simulink model "adarbha_hw6_sim"  (Simulink 7.7)
settings: Solver=ode1  StartTime=0.0  StopTime=max(Time)  FixedStep=0.5  RelTol=1e-5
InitFcn:
  | adarbha_hw6
values from neighbouring files (symbols this model uses):
  Area = 2.7    [adarbha_hw6.m]    (also in hw6.m; hw6_code.m)
  Cd = 0.44    [adarbha_hw6.m]    (also in hw6.m; hw6_code.m)
  density = 1.224    [adarbha_hw6.m]    (also in hw6.m; hw6_code.m)
  Q = 20    [adarbha_hw6.m]    (also in hw6_code.m)
  R_batt = 0.1    [adarbha_hw6.m]    (also in hw6_code.m)
  radius_wheel_m = 0.41    [adarbha_hw6.m]    (also in hw6.m; hw6_code.m)
  rpm = 1:5000    [adarbha_hw6.m]    (also in hw6.m; hw6_code.m)
  Time = xlsread('Malibu_20100929_highway_Baseline','A:A')    [adarbha_hw6.m]    (also in hw6.m; hw6_code.m)
  time_s = time_scale*100    [adarbha_hw6.m]    (also in hw6.m; hw6_code.m)
  V_o = 300    [adarbha_hw6.m]    (also in hw6_code.m)
  vel_m_s = M_number*3    [adarbha_hw6.m]    (also in hw6.m; hw6_code.m)
  Velocity_kph = xlsread('Malibu_20100929_highway_Baseline','B:B')    [adarbha_hw6.m]    (also in hw6.m; hw6_code.m)
  weight_N = 16000    [adarbha_hw6.m]    (also in hw6.m; hw6_code.m)
undefined symbols (not defined in the file or in its folder): torque
libraries: simulink x3
settings Model: Creator=Arjun  LastModifiedBy=Arjun
settings DataIOCC: SignalLogging=off
settings DebuggingCC: AlgebraicLoopMsg=none

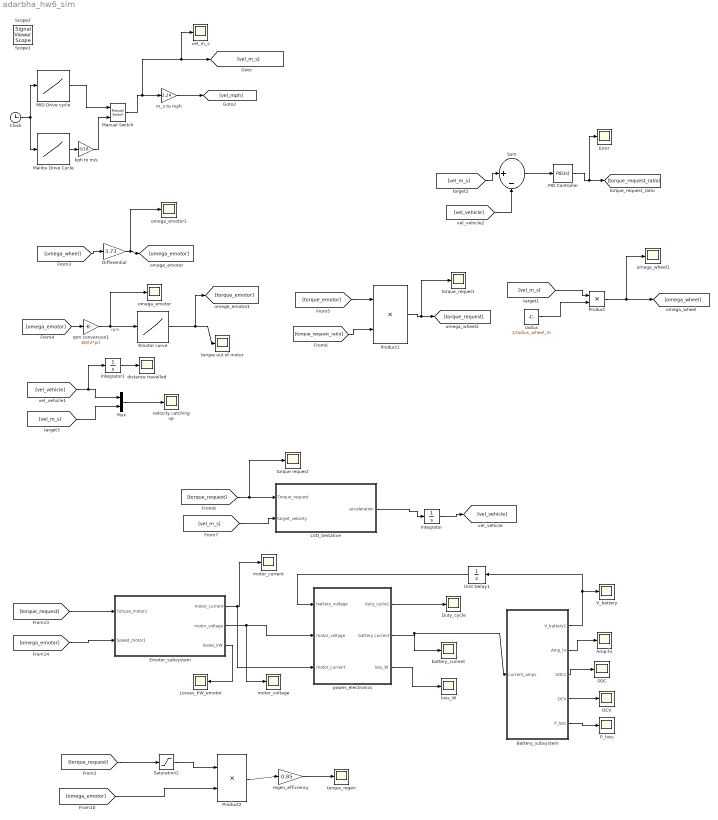
== system adarbha_hw6_sim ==
  note: rpm
  Amp-hr : Scope
      settings: SaveName=ScopeData23
  Battery_subsystem : Subsystem
  Clock : Clock
      settings: Decimation=10
  Differential : Gain  Gain=3.73
  Duty_cycle : Scope
      settings: SaveName=ScopeData22
  Emotor curve : Lookup_n-D  NumberOfTableDimensions=1  BreakpointsForDimension1=rpm  Table=torque  RndMeth=Simplest  InputSameDT=on
  Emotor_subsystem : Subsystem
  Error : Scope
      settings: SaveName=ScopeData17
  Integrator : Integrator
  Integrator1 : Integrator
  LVD_tentative : Subsystem
  Losses_kW_emotor : Scope
      settings: SaveName=ScopeData19
  MID Drive cycle : Lookup_n-D  NumberOfTableDimensions=1  BreakpointsForDimension1=time_s  Table=vel_m_s  RndMeth=Simplest  InputSameDT=on
  Malibu Drive Cycle : Lookup_n-D  NumberOfTableDimensions=1  BreakpointsForDimension1=Time  Table=Velocity_kph  RndMeth=Simplest  InputSameDT=on
  Manual Switch : simulink/Signal Routing/Manual Switch  SystemSampleTime=-1  sw=0  action=0  varsize=off
  Mux : Mux  Inputs=2
  OCV : Scope
      settings: SaveName=ScopeData31
  PID Controller : simulink/Continuous/PID Controller  SystemSampleTime=-1  Controller=PID  TimeDomain=Continuous-time  SampleTime=1  IntegratorMethod=Forward Euler  FilterMethod=Forward Euler  Form=Parallel  P=1  I=1  D=0  N=100  InitialConditionSource=internal  InitialConditionForIntegrator=0  InitialConditionForFilter=0  ExternalReset=none  LimitOutput=off  UpperSaturationLimit=inf  LowerSaturationLimit=-inf  LinearizeAsGain=off  AntiWindupMode=none  Kb=1  TrackingMode=off  Kt=1  PParamMin=[]  PParamMax=[]  IParamMin=[]  IParamMax=[]  DParamMin=[]  DParamMax=[]  NParamMin=[]  NParamMax=[]  KbParamMin=[]  KbParamMax=[]  KtParamMin=[]  KtParamMax=[]  POutMin=[]  POutMax=[]  IOutMin=[]  IOutMax=[]  DOutMin=[]  DOutMax=[]  NOutMin=[]  NOutMax=[]  KbOutMin=[]  KbOutMax=[]  KtOutMin=[]  KtOutMax=[]  IntegratorOutMin=[]  IntegratorOutMax=[]  FilterOutMin=[]  FilterOutMax=[]  SumOutMin=[]  SumOutMax=[]  SumI1OutMin=[]  SumI1OutMax=[]  SumI2OutMin=[]  SumI2OutMax=[]  SumI3OutMin=[]  SumI3OutMax=[]  SumDOutMin=[]  SumDOutMax=[]  SaturationOutMin=[]  SaturationOutMax=[]  IntegratorContinuousStateAttributes=''  IntegratorStateMustResolveToSignalObject=off  IntegratorRTWStateStorageClass=Auto  FilterContinuousStateAttributes=''  FilterStateMustResolveToSignalObject=off  FilterRTWStateStorageClass=Auto
  P_loss : Scope
      settings: SaveName=ScopeData33
  Product : Product  RndMeth=Zero
  Product1 : Product  RndMeth=Zero
  Product2 : Product  RndMeth=Zero
  SOC : Scope
      settings: SaveName=ScopeData28
  Saturation2 : Saturate  UpperLimit=0  LowerLimit=-Inf
  Sum : Sum  Inputs=|+-
  Unit Delay1 : UnitDelay  SampleTime=-1
  V_battery : Scope
      settings: TimeRange=500  YMin=-50  YMax=300  SaveName=ScopeData29
  battery_current : Scope
      settings: SaveName=ScopeData24
  distance travelled : Scope
      settings: SaveName=ScopeData25
  kph to m/s : Gain  Gain=5/18
  loss_W : Scope
      settings: SaveName=ScopeData20
  m_s to mph : Gain  Gain=2.24
  motor_current : Scope
      settings: SaveName=ScopeData11
  motor_voltage : Scope
      settings: SaveName=ScopeData26
  omega_emotor : Scope
      settings: SaveName=ScopeData7
  omega_emotor1 : Scope
      settings: SaveName=ScopeData32
  omega_wheel1 : Scope
      settings: SaveName=ScopeData4
  power_electronics : Subsystem
  radius : Constant  Value=1/radius_wheel_m
  regen_efficiency : Gain  Gain=0.85
  rpm conversion1 : Gain  Gain=60/(2*pi)
  torque out of motor : Scope
      settings: SaveName=ScopeData8
  torque request : Scope
      settings: SaveName=ScopeData12
  torque_regen : Scope
      settings: SaveName=ScopeData16
  torque_request : Scope
      settings: SaveName=ScopeData6
  vel_m_s : Scope
      settings: SaveName=ScopeData21
  velocity catching up : Scope
      settings: TimeRange=765.8724058416602  YMin=-1e+049  YMax=9.000000000000001e+049  SaveName=ScopeData18
  Scope1 : SignalViewerScope  IOType=viewer  NumInputPorts=5  RefreshTime=0.035000
  Scope2 : SignalViewerScope  IOType=viewer  RefreshTime=0.035000
  wires:
  m_s to mph/1 -> [vel_mph]
  Clock/1 -> MID Drive cycle/1, Malibu Drive Cycle/1
  [vel_m_s] -> Product/1
  Product/1 -> [omega_wheel], omega_wheel1/1
  radius/1 -> Product/2
  [torque_emotor] -> Product1/1
  [torque_request_ratio] -> Product1/2
  Product1/1 -> [torque_request], torque_request/1
  [omega_wheel] -> Differential/1
  Differential/1 -> [omega_emotor], omega_emotor1/1
  [omega_emotor] -> rpm conversion1/1
  Emotor curve/1 -> torque out of motor/1, [torque_emotor]
  [vel_m_s] -> LVD_tentative/2(target_velocity)
  [torque_request] -> LVD_tentative/1(Torque_request), torque request/1
  Integrator/1 -> [vel_vehicle]
  LVD_tentative/1(acceleration) -> Integrator/1
  [vel_m_s] -> Sum/1
  [vel_vehicle] -> Sum/2
  [vel_m_s] -> Mux/2
  [vel_vehicle] -> Mux/1, Integrator1/1
  Mux/1 -> velocity catching up/1
  MID Drive cycle/1 -> Manual Switch/1
  Manual Switch/1 -> m_s to mph/1, [vel_m_s], vel_m_s/1
  Malibu Drive Cycle/1 -> kph to m/s/1
  kph to m/s/1 -> Manual Switch/2
  Integrator1/1 -> distance travelled/1
  power_electronics/2(battery current) -> battery_current/1, Battery_subsystem/1(current_amps)
  Battery_subsystem/1(V_battery1) -> V_battery/1, Unit Delay1/1
  Battery_subsystem/3(SOC1) -> SOC/1
  [torque_request] -> Saturation2/1
  Saturation2/1 -> Product2/1
  [omega_emotor] -> Product2/2
  Product2/1 -> regen_efficiency/1
  regen_efficiency/1 -> torque_regen/1
  power_electronics/3(loss_W) -> loss_W/1
  power_electronics/1(duty_cycle1) -> Duty_cycle/1
  Battery_subsystem/2(Amp_hr) -> Amp-hr/1
  Battery_subsystem/4(OCV) -> OCV/1
  Battery_subsystem/5(P_loss) -> P_loss/1
  rpm conversion1/1 -> Emotor curve/1, omega_emotor/1
  Unit Delay1/1 -> power_electronics/1(battery_voltage)
  Emotor_subsystem/3(losses_kW) -> Losses_kW_emotor/1
  Emotor_subsystem/2(motor_voltage) -> power_electronics/2(motor_voltage), motor_voltage/1
  Emotor_subsystem/1(motor_current) -> motor_current/1, power_electronics/3(motor_current)
  [torque_request] -> Emotor_subsystem/1(Torque_motor1)
  [omega_emotor] -> Emotor_subsystem/2(Speed_motor1)
  Sum/1 -> PID Controller/1
  PID Controller/1 -> [torque_request_ratio], Error/1

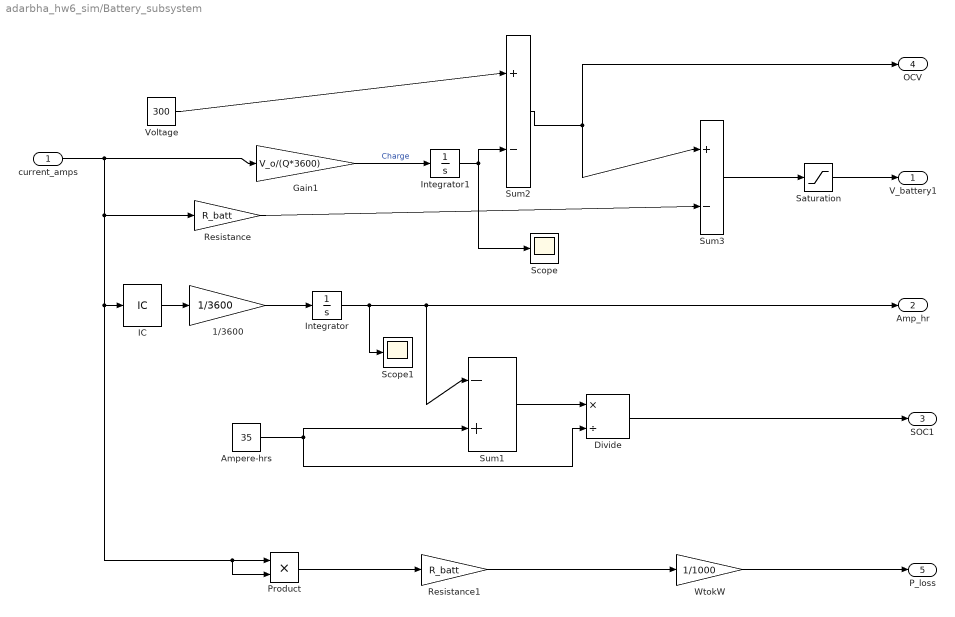
== system adarbha_hw6_sim/Battery_subsystem ==
  current_amps : Inport
  1/3600 : Gain  Gain=1/3600
  Ampere-hrs : Constant  Value=35
  Divide : Product  Inputs=*/
  Gain1 : Gain  Gain=V_o/(Q*3600)
  IC : InitialCondition  Value=0.1
  Integrator : Integrator  InitialCondition=0.1  LimitOutput=on  UpperSaturationLimit=20  LowerSaturationLimit=0
  Integrator1 : Integrator  LimitOutput=on  UpperSaturationLimit=300  LowerSaturationLimit=0
  Product : Product  RndMeth=Zero
  Resistance : Gain  Gain=R_batt
  Resistance1 : Gain  Gain=R_batt
  Saturation : Saturate  UpperLimit=300  LowerLimit=1  ZeroCross=off
  Scope : Scope
  Scope1 : Scope
      settings: SaveName=ScopeData3
  Sum1 : Sum  Inputs=|-+
  Sum2 : Sum  Inputs=|+-
  Sum3 : Sum  Inputs=|+-
  Voltage : Constant  Value=300
  WtokW : Gain  Gain=1/1000
  V_battery1 : Outport
  Amp_hr : Outport  Port=2
  SOC1 : Outport  Port=3
  OCV : Outport  Port=4
  P_loss : Outport  Port=5
  wires:
  Gain1/1 -> Integrator1/1  "Charge"
  Integrator1/1 -> Sum2/2, Scope/1
  Resistance/1 -> Sum3/2
  Ampere-hrs/1 -> Sum1/2, Divide/2
  Sum1/1 -> Divide/1
  Divide/1 -> SOC1/1
  current_amps/1 -> Gain1/1, Product/1, Product/2, IC/1, Resistance/1
  Product/1 -> Resistance1/1
  Resistance1/1 -> WtokW/1
  1/3600/1 -> Integrator/1
  Integrator/1 -> Amp_hr/1, Sum1/1, Scope1/1
  Sum3/1 -> Saturation/1
  Voltage/1 -> Sum2/1
  Sum2/1 -> Sum3/1, OCV/1
  Saturation/1 -> V_battery1/1
  WtokW/1 -> P_loss/1
  IC/1 -> 1/3600/1

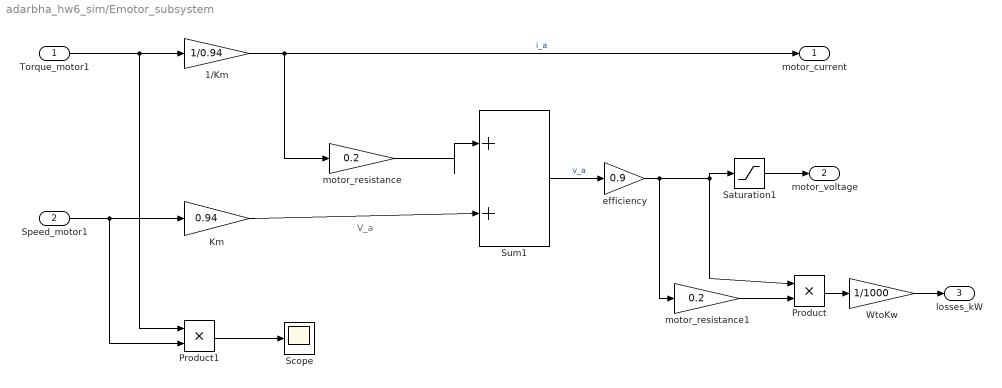
== system adarbha_hw6_sim/Emotor_subsystem ==
  note: V_a
  Torque_motor1 : Inport
  Speed_motor1 : Inport  Port=2
  1/Km : Gain  Gain=1/0.94
  Km : Gain  Gain=0.94
  Product : Product  RndMeth=Zero
  Product1 : Product  RndMeth=Zero
  Saturation1 : Saturate  UpperLimit=300  LowerLimit=0
  Scope : Scope
      settings: SaveName=ScopeData30
  Sum1 : Sum  Inputs=|++
  WtoKw : Gain  Gain=1/1000
  efficiency : Gain  Gain=0.9
  motor_resistance : Gain  Gain=0.2
  motor_resistance1 : Gain  Gain=0.2
  motor_current : Outport
  motor_voltage : Outport  Port=2
  losses_kW : Outport  Port=3
  wires:
  Torque_motor1/1 -> 1/Km/1, Product1/1
  Speed_motor1/1 -> Km/1, Product1/2
  Km/1 -> Sum1/2
  1/Km/1 -> motor_resistance/1, motor_current/1  "i_a"
  motor_resistance/1 -> Sum1/1
  motor_resistance1/1 -> Product/2
  Product/1 -> WtoKw/1
  WtoKw/1 -> losses_kW/1
  Saturation1/1 -> motor_voltage/1
  Product1/1 -> Scope/1
  efficiency/1 -> motor_resistance1/1, Product/1, Saturation1/1
  Sum1/1 -> efficiency/1  "v_a"

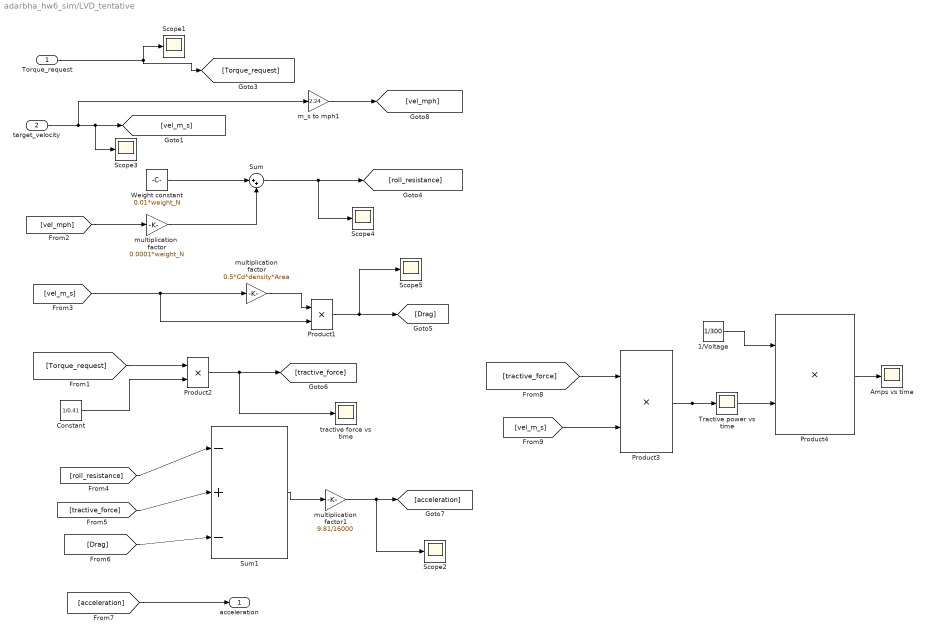
== system adarbha_hw6_sim/LVD_tentative ==
  Torque_request : Inport
  target_velocity : Inport  Port=2
  1/Voltage : Constant  Value=1/300
  Amps vs time : Scope
      settings: SaveName=ScopeData15
  Constant : Constant  Value=1/0.41
  Product{1..4} (4 alike) : Product  RndMeth=Zero
  Scope{1..5} (5 alike) : Scope
      Scope1 settings: SaveName=ScopeData5
      Scope2 settings: SaveName=ScopeData6
      Scope3 settings: SaveName=ScopeData8
      Scope4 settings: SaveName=ScopeData9
      Scope5 settings: SaveName=ScopeData10
  Sum : Sum  Inputs=|++
  Sum1 : Sum  Inputs=|-+-
  Tractive power vs time : Scope
      settings: SaveName=ScopeData14
  Weight constant : Constant  Value=0.01*weight_N
  m_s to mph1 : Gain  Gain=2.24
  multiplication  factor : Gain  Gain=0.0001*weight_N
  multiplication factor : Gain  Gain=0.5*Cd*density*Area
  multiplication factor1 : Gain  Gain=9.81/16000
  tractive force vs time : Scope
      settings: SaveName=ScopeData13
  acceleration : Outport
  wires:
  Weight constant/1 -> Sum/1
  multiplication  factor/1 -> Sum/2
  Sum/1 -> [roll_resistance], Scope4/1
  [vel_mph] -> multiplication  factor/1
  multiplication factor/1 -> Product1/1
  [vel_m_s] -> multiplication factor/1, Product1/2
  Product1/1 -> [Drag], Scope5/1
  [Torque_request] -> Product2/1
  Constant/1 -> Product2/2
  Product2/1 -> [tractive_force], tractive force vs time/1
  [roll_resistance] -> Sum1/1
  [tractive_force] -> Sum1/2
  [Drag] -> Sum1/3
  Sum1/1 -> multiplication factor1/1
  multiplication factor1/1 -> [acceleration], Scope2/1
  Torque_request/1 -> [Torque_request], Scope1/1
  target_velocity/1 -> m_s to mph1/1, [vel_m_s], Scope3/1
  m_s to mph1/1 -> [vel_mph]
  [acceleration] -> acceleration/1
  [tractive_force] -> Product3/1
  [vel_m_s] -> Product3/2
  Product3/1 -> Tractive power vs time/1, Product4/2
  1/Voltage/1 -> Product4/1
  Product4/1 -> Amps vs time/1

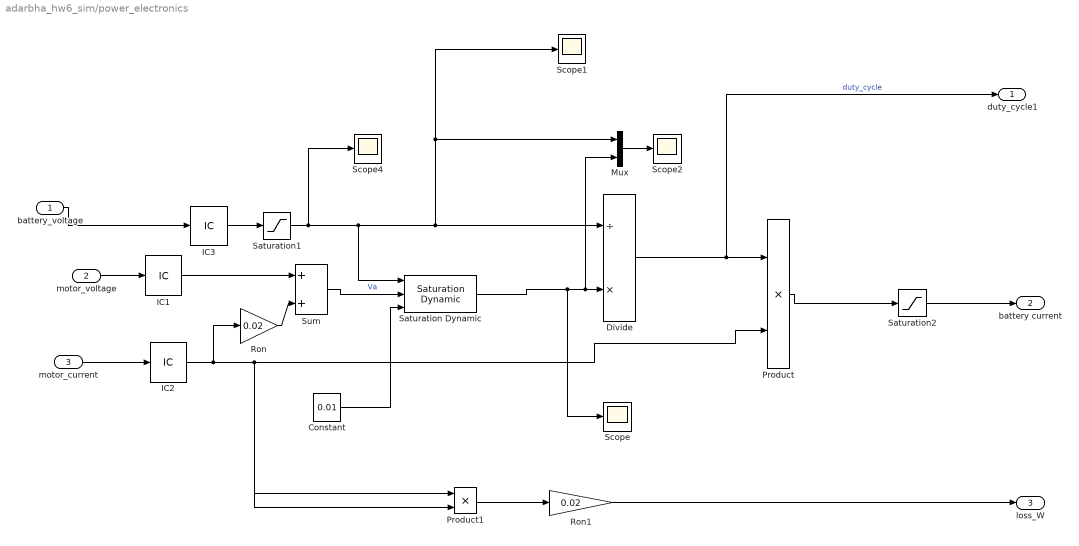
== system adarbha_hw6_sim/power_electronics ==
  battery_voltage : Inport
  motor_voltage : Inport  Port=2
  motor_current : Inport  Port=3
  Constant : Constant  Value=0.01
  Divide : Product  Inputs=/*
  IC1 : InitialCondition  Value=0.01
  IC2 : InitialCondition  Value=0.01
  IC3 : InitialCondition
  Mux : Mux  Inputs=2
  Product : Product  RndMeth=Zero
  Product1 : Product  RndMeth=Zero
  Ron : Gain  Gain=0.02
  Ron1 : Gain  Gain=0.02
  Saturation Dynamic : simulink/Discontinuities/Saturation Dynamic  SystemSampleTime=-1  OutMin=[]  OutMax=[]  OutDataTypeStr=Inherit: Same as second input  OutDataType=fixdt(1, 16)  OutScaling=2^-10  DoSatur=off
  Saturation1 : Saturate  UpperLimit=300  LowerLimit=1  ZeroCross=off
  Saturation2 : Saturate  UpperLimit=100  LowerLimit=-400  ZeroCross=off
  Scope{,1..2,4} (4 alike) : Scope
      Scope1 settings: SaveName=ScopeData2
      Scope2 settings: SaveName=ScopeData27
      Scope4 settings: SaveName=ScopeData35
  Sum : Sum  Inputs=|++
  duty_cycle1 : Outport
  battery current : Outport  Port=2
  loss_W : Outport  Port=3
  wires:
  battery_voltage/1 -> IC3/1
  motor_voltage/1 -> IC1/1
  motor_current/1 -> IC2/1
  Divide/1 -> Product/1, duty_cycle1/1  "duty_cycle"
  Product1/1 -> Ron1/1
  Product/1 -> Saturation2/1
  Ron1/1 -> loss_W/1
  Ron/1 -> Sum/2
  IC1/1 -> Sum/1
  IC2/1 -> Product/2, Product1/1, Product1/2, Ron/1
  Saturation2/1 -> battery current/1
  Mux/1 -> Scope2/1
  IC3/1 -> Saturation1/1
  Saturation1/1 -> Scope4/1, Divide/1, Scope1/1, Mux/1, Saturation Dynamic/1
  Saturation Dynamic/1 -> Scope/1, Divide/2, Mux/2
  Sum/1 -> Saturation Dynamic/2  "Va"
  Constant/1 -> Saturation Dynamic/3
